simulink model "sim4_5"  (R2022a)
settings: Solver=FixedStepAuto  StartTime=0.0  StopTime=120  FixedStep=0.001  MaxStep=0.002  RelTol=1e-3
libraries: fl_lib x16, nesl_utility x7, dspadpt3 x6, dsparch4 x3
settings Model: Creator=targi  LastModifiedBy=targi

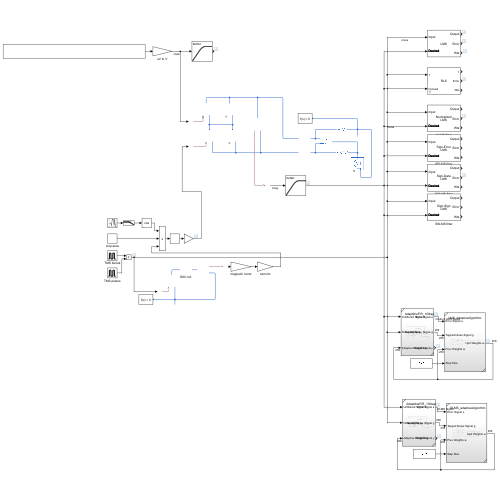
[thumbnail: Simulink's stored preview of the top-level diagram]
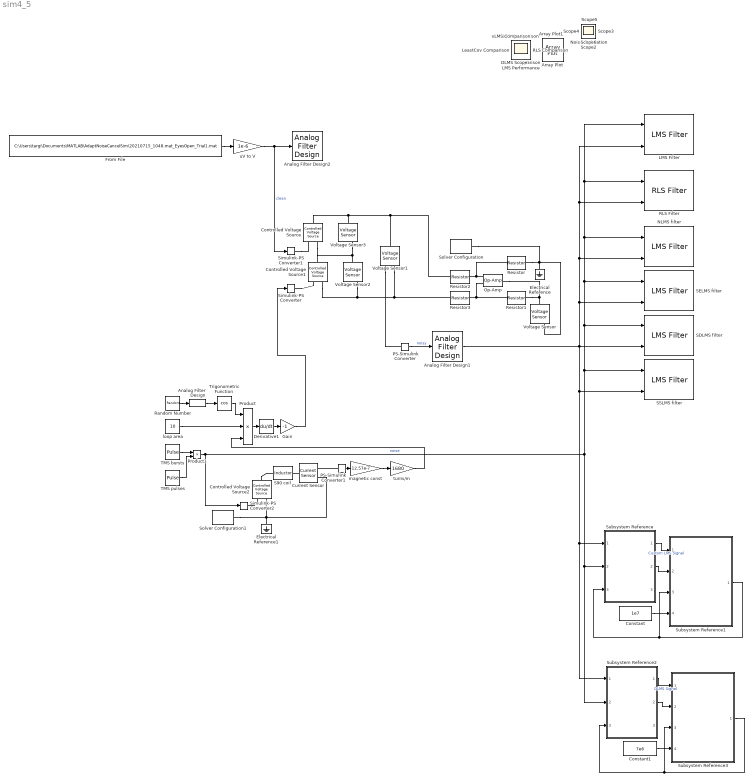
== system sim4_5 ==
  Analog Filter Design : dsparch4/Analog Filter Design  method=Butterworth  filttype=Lowpass  N=8  Wlo=100  Whi=80  Rp=2  Rs=40
  Analog Filter Design1 : dsparch4/Analog Filter Design  method=Butterworth  filttype=Highpass  N=2  Wlo=10  Whi=80  Rp=2  Rs=40
  Analog Filter Design2 : dsparch4/Analog Filter Design  method=Butterworth  filttype=Highpass  N=2  Wlo=10  Whi=80  Rp=2  Rs=40
  Constant : Constant  Value=1e7
  Constant1 : Constant  Value=7e6
  Controlled Voltage Source : fl_lib/Electrical/Electrical Sources/Controlled Voltage Source
      settings: SourceProductBaseCode=PW,SS,VE
  Controlled Voltage Source1 : fl_lib/Electrical/Electrical Sources/Controlled Voltage Source
      settings: SourceProductBaseCode=PW,SS,VE
  Controlled Voltage Source2 : fl_lib/Electrical/Electrical Sources/Controlled Voltage Source
      settings: SourceProductBaseCode=PW,SS,VE
  Current Sensor : fl_lib/Electrical/Electrical Sensors/Current Sensor
      settings: SourceProductBaseCode=PW,SS,VE
  Derivative1 : Derivative
  Electrical Reference : fl_lib/Electrical/Electrical Elements/Electrical Reference
      settings: SourceProductBaseCode=PW,SS,VE
  Electrical Reference1 : fl_lib/Electrical/Electrical Elements/Electrical Reference
      settings: SourceProductBaseCode=PW,SS,VE
  From File : FromFile  FileName=C:\Users\targi\Documents\MATLAB\AdaptNoiseCancelSim\20210715_1048.mat_EyesOpen_Trial1.mat
  Gain : Gain  Gain=-1
  LMS Filter : dspadpt3/LMS Filter  Algo=LMS  L=256  stepflag=Dialog  mu=1e7  leakage=1  ic=0  Adapt=off  resetflag=None  weights=on  addnparflag=off  roundingMode=Floor  overflowMode=off  firstCoeffMode=Binary point scaling  firstCoeffWordLength=16  firstCoeffFracLength=15
      settings: SourceProductBaseCode=DS
  NLMS filter : dspadpt3/LMS Filter  Algo=Normalized LMS  L=256  stepflag=Dialog  mu=1  leakage=1.0  ic=0  Adapt=off  resetflag=None  weights=on  addnparflag=off  roundingMode=Floor  overflowMode=off
      settings: SourceProductBaseCode=DS
  Op-Amp : fl_lib/Electrical/Electrical Elements/Op-Amp  outI_specify=off  outI_priority=None  outI=0 A  outI_nominal_specify=off  outI_nominal_unit=A  outI_nominal_value=1
      settings: SourceProductBaseCode=PW,SS,VE
  PS-Simulink Converter : nesl_utility/PS-Simulink Converter  PhysicalDomain=network_engine_domain  SubClassName=ps_output  LeftPortType=input  RightPortType=output  PseudoPeriodic=off  Frequencies=[]  VectorFormat=inherit  Unit=inherit  AffineConversion=off
      settings: SourceProductBaseCode=SS,PW,VE
  PS-Simulink Converter1 : nesl_utility/PS-Simulink Converter  PhysicalDomain=network_engine_domain  SubClassName=ps_output  LeftPortType=input  RightPortType=output  PseudoPeriodic=off  Frequencies=[]  VectorFormat=inherit  Unit=inherit  AffineConversion=off
      settings: SourceProductBaseCode=SS,PW,VE
  Product : Product  Inputs=3
  Product1 : Product
  RLS Filter : dspadpt3/RLS Filter  L=32  lambdaflag=Dialog  lambda=1  addnparflag=on  ic=0  delta=0.1  Adapt=off  resetflag=None  weights=on
      settings: SourceProductBaseCode=DS
  Random Number : RandomNumber  Variance=.15
  Resistor : fl_lib/Electrical/Electrical Elements/Resistor  R=100 Ohm  i_specify=off  i_priority=None  i=0 A  i_nominal_specify=off  i_nominal_unit=A  i_nominal_value=1  v_specify=off  v_priority=None  v=0 V  v_nominal_specify=off  v_nominal_unit=V  v_nominal_value=1
      settings: SourceProductBaseCode=PW,SS,VE
  Resistor1 : fl_lib/Electrical/Electrical Elements/Resistor  R=100 Ohm  i_specify=off  i_priority=None  i=0 A  i_nominal_specify=off  i_nominal_unit=A  i_nominal_value=1  v_specify=off  v_priority=None  v=0 V  v_nominal_specify=off  v_nominal_unit=V  v_nominal_value=1
      settings: SourceProductBaseCode=PW,SS,VE
  Resistor2 : fl_lib/Electrical/Electrical Elements/Resistor  R=1 Ohm  i_specify=off  i_priority=None  i=0 A  i_nominal_specify=off  i_nominal_unit=A  i_nominal_value=1  v_specify=off  v_priority=None  v=0 V  v_nominal_specify=off  v_nominal_unit=V  v_nominal_value=1
      settings: SourceProductBaseCode=PW,SS,VE
  Resistor3 : fl_lib/Electrical/Electrical Elements/Resistor  R=1 Ohm  i_specify=off  i_priority=None  i=0 A  i_nominal_specify=off  i_nominal_unit=A  i_nominal_value=1  v_specify=off  v_priority=None  v=0 V  v_nominal_specify=off  v_nominal_unit=V  v_nominal_value=1
      settings: SourceProductBaseCode=PW,SS,VE
  S90 coil : fl_lib/Electrical/Electrical Elements/Inductor  l=23.47 uH  r=.01 Ohm  g=1e-9 1/Ohm  i_specify=off  i_priority=None  i=0 A  i_nominal_specify=off  i_nominal_unit=A  i_nominal_value=1  v_specify=off  v_priority=None  v=0 V  v_nominal_specify=off  v_nominal_unit=V  v_nominal_value=1  i_L_specify=off  i_L_priority=High  i_L=0 A  i_L_nominal_specify=off  i_L_nominal_unit=A  i_L_nominal_value=1
      settings: SourceProductBaseCode=PW,SS,VE
  SDLMS filter : dspadpt3/LMS Filter  Algo=Sign-Data LMS  L=256  stepflag=Dialog  mu=1e3  leakage=1.0  ic=0  Adapt=off  resetflag=None  weights=on  addnparflag=off  roundingMode=Floor  overflowMode=off
      settings: SourceProductBaseCode=DS
  SELMS filter : dspadpt3/LMS Filter  Algo=Sign-Error LMS  L=256  stepflag=Dialog  mu=1e4  leakage=1.0  ic=0  Adapt=off  resetflag=None  weights=on  addnparflag=off  roundingMode=Floor  overflowMode=off
      settings: SourceProductBaseCode=DS
  SSLMS filter : dspadpt3/LMS Filter  Algo=Sign-Sign LMS  L=256  stepflag=Dialog  mu=1  leakage=1.0  ic=0  Adapt=off  resetflag=None  weights=on  addnparflag=off  roundingMode=Floor  overflowMode=off
      settings: SourceProductBaseCode=DS
  Simulink-PS Converter : nesl_utility/Simulink-PS Converter  PhysicalDomain=network_engine_domain  SubClassName=ps_input  LeftPortType=input  RightPortType=output  PseudoPeriodic=off  Frequencies=[]  NoiseDistribution=none  NoiseParameters=[]  Unit=1  AffineConversion=off  FilteringAndDerivatives=provide  SimscapeFilterOrder=1  InputFilterTimeConstant=0.001  UdotUserProvided=0
      settings: SourceProductBaseCode=SS,PW,VE
  Simulink-PS Converter1 : nesl_utility/Simulink-PS Converter  PhysicalDomain=network_engine_domain  SubClassName=ps_input  LeftPortType=input  RightPortType=output  PseudoPeriodic=off  Frequencies=[]  NoiseDistribution=none  NoiseParameters=[]  Unit=1  AffineConversion=off  FilteringAndDerivatives=provide  SimscapeFilterOrder=1  InputFilterTimeConstant=0.001  UdotUserProvided=0
      settings: SourceProductBaseCode=SS,PW,VE
  Simulink-PS Converter2 : nesl_utility/Simulink-PS Converter  PhysicalDomain=network_engine_domain  SubClassName=ps_input  LeftPortType=input  RightPortType=output  PseudoPeriodic=off  Frequencies=[]  NoiseDistribution=none  NoiseParameters=[]  Unit=1  AffineConversion=off  FilteringAndDerivatives=provide  SimscapeFilterOrder=1  InputFilterTimeConstant=0.001  UdotUserProvided=0
      settings: SourceProductBaseCode=SS,PW,VE
  Solver Configuration : nesl_utility/Solver Configuration  PhysicalDomain=network_engine_domain  SubClassName=solver  LeftPortType=input  RightPortType=generic  Tones=[]  Harmonics=[]  SimulateNoise=off  Profile=off  UseLocalSampling=off  EnableSwitchedLinearOptims=on  FrequencyDomain=off  UseCCode=off  RelTol=0.001  AbsTol=0.001  MinStep=1e-09  ToWorkspace=off  RevertToSquareIcSolve=off  NumHomotopyIterations=100  PhasorMode=off  PhasorModeNumHarmonics=1  IndexReductionMethod=DerivativeReplacement  DoDC=off  ResidualTolerance=1e-09  UseLocalSolver=off  LocalSolverChoice=NE_BACKWARD_EULER_ADVANCER  LocalSolverSampleTime=0.001  DoFixedCost=off  MaxNonlinIter=3  MaxModeIter=2  ComputeImpulses=off  ImpulseIterations=2  LinearAlgebra=auto  LinearAlgebraNumThread=0  EquationFormulation=NE_TIME_EF  DelaysMemoryBudget=1024  AutomaticFiltering=on  FilteringTimeConstant=0.001  PartitionStorageMethod=AS_NEEDED  PartitionMemoryBudget=1024  PartitionMethod=ROBUST
      settings: SourceProductBaseCode=SS,PW,VE
  Solver Configuration1 : nesl_utility/Solver Configuration  PhysicalDomain=network_engine_domain  SubClassName=solver  LeftPortType=input  RightPortType=generic  Tones=[]  Harmonics=[]  SimulateNoise=off  Profile=off  UseLocalSampling=off  EnableSwitchedLinearOptims=on  FrequencyDomain=off  UseCCode=off  RelTol=0.001  AbsTol=0.001  MinStep=1e-09  ToWorkspace=off  RevertToSquareIcSolve=off  NumHomotopyIterations=100  PhasorMode=off  PhasorModeNumHarmonics=1  IndexReductionMethod=DerivativeReplacement  DoDC=off  ResidualTolerance=1e-09  UseLocalSolver=off  LocalSolverChoice=NE_BACKWARD_EULER_ADVANCER  LocalSolverSampleTime=0.001  DoFixedCost=off  MaxNonlinIter=3  MaxModeIter=2  ComputeImpulses=off  ImpulseIterations=2  LinearAlgebra=auto  LinearAlgebraNumThread=0  EquationFormulation=NE_TIME_EF  DelaysMemoryBudget=1024  AutomaticFiltering=on  FilteringTimeConstant=0.001  PartitionStorageMethod=AS_NEEDED  PartitionMemoryBudget=1024  PartitionMethod=ROBUST
      settings: SourceProductBaseCode=SS,PW,VE
  Subsystem Reference : Subsystem  ReferencedSubsystem=AdaptibleFIR_100taps
  Subsystem Reference1 : Subsystem  ReferencedSubsystem=LMS_adaptiveAlgorithm
  Subsystem Reference2 : Subsystem  ReferencedSubsystem=AdaptibleFIR_100taps
  Subsystem Reference3 : Subsystem  ReferencedSubsystem=DLMS_adaptiveAlgorithm
  TMS bursts : DiscretePulseGenerator  PulseType=Time based  Period=.02  PulseWidth=5
  TMS pulses : DiscretePulseGenerator  PulseType=Time based  Amplitude=1e-4  Period=.2  PulseWidth=29
  Trigonometric Function : Trigonometry  Operator=cos
  Voltage Sensor{,1..3} (4 alike) : fl_lib/Electrical/Electrical Sensors/Voltage Sensor
      settings: SourceProductBaseCode=PW,SS,VE
  loop area : Constant  Value=10
  magnetic const : Gain  Gain=12.57e-7
  turns/m : Gain  Gain=1680
  uV to V : Gain  Gain=1e-6
  Array Plot : ArrayPlot  IOType=viewer  WindowPosition=[698.000000,462.000000,800.000000,500.000000,]  Visible=on  IsFloating=on  ScopeFrameLocation=window  YLimits=[-35.4102,168.2872]  DefaultConfigurationName=dsp.scopes.ArrayPlotBlockSpecification
  Array Plot1 : ArrayPlot  IOType=viewer  WindowPosition=[44.000000,61.000000,800.000000,500.000000,]  Visible=on  IsFloating=on  ScopeFrameLocation=window  YLimits=[-41.2548,164.9494]  DefaultConfigurationName=dsp.scopes.ArrayPlotBlockSpecification
  DLMS Comparison : Scope
  LMS Comparison : Scope
  LMS Performance : Scope
  LeastCov Comparison : Scope
  Noise Estimation : Scope
  RLS Comparison : Scope
  Scope{,1..6} (7 alike) : Scope
  vLMS Comparison : Scope
  wires:
  Product1/1 -> Simulink-PS Converter2/1, RLS Filter/1, LMS Filter/1, NLMS filter/1, SELMS filter/1, SDLMS filter/1, SSLMS filter/1, Subsystem Reference2/2, Subsystem Reference/2  "noise"
  uV to V/1 -> Analog Filter Design2/1, Simulink-PS Converter1/1  "clean"
  PS-Simulink Converter/1 -> Analog Filter Design1/1  "noisy"
  Subsystem Reference/1 -> Subsystem Reference1/1  "Custom LMS Signal"
  Subsystem Reference/2 -> Subsystem Reference1/2
  Subsystem Reference1/1 -> Subsystem Reference1/3, Subsystem Reference/3
  Constant/1 -> Subsystem Reference1/4
  Constant1/1 -> Subsystem Reference3/4
  Subsystem Reference2/2 -> Subsystem Reference3/2
  Subsystem Reference2/1 -> Subsystem Reference3/1  "DLMS Signal"
  Subsystem Reference3/1 -> Subsystem Reference3/3, Subsystem Reference2/3
  loop area/1 -> Product/2
  Trigonometric Function/1 -> Product/1
  Product/1 -> Derivative1/1
  Derivative1/1 -> Gain/1
  Gain/1 -> Simulink-PS Converter/1
  Random Number/1 -> Analog Filter Design/1
  Analog Filter Design/1 -> Trigonometric Function/1
  TMS bursts/1 -> Product1/1
  TMS pulses/1 -> Product1/2
  From File/1 -> uV to V/1
  PS-Simulink Converter1/1 -> magnetic const/1
  magnetic const/1 -> turns/m/1
  turns/m/1 -> Product/3
  Analog Filter Design1/1 -> Subsystem Reference2/1, Subsystem Reference/1, SSLMS filter/2, LMS Filter/2, RLS Filter/2, NLMS filter/2, SELMS filter/2, SDLMS filter/2
  connections:
  Resistor2/RConn1 -- Resistor/LConn1 -- Op-Amp/LConn1
  Resistor1/LConn1 -- Op-Amp/LConn2 -- Resistor3/RConn1
  Op-Amp/RConn1 -- Resistor1/RConn1 -- Voltage Sensor/LConn1
  Resistor/RConn1 -- Solver Configuration/RConn1 -- Electrical Reference/LConn1 -- Voltage Sensor/RConn2
  Resistor2/LConn1 -- Controlled Voltage Source/LConn1 -- Voltage Sensor3/LConn1 -- Voltage Sensor1/LConn1
  Voltage Sensor3/RConn2 -- Controlled Voltage Source/RConn2 -- Controlled Voltage Source1/LConn1 -- Voltage Sensor2/LConn1
  Voltage Sensor1/RConn2 -- Controlled Voltage Source1/RConn2 -- Voltage Sensor2/RConn2 -- Resistor3/LConn1
  Simulink-PS Converter/RConn1 -- Controlled Voltage Source1/RConn1
  Simulink-PS Converter1/RConn1 -- Controlled Voltage Source/RConn1
  Voltage Sensor1/RConn1 -- PS-Simulink Converter/LConn1
  Simulink-PS Converter2/RConn1 -- Controlled Voltage Source2/RConn1
  S90 coil/LConn1 -- Controlled Voltage Source2/LConn1
  S90 coil/RConn1 -- Current Sensor/LConn1
  Current Sensor/RConn2 -- Controlled Voltage Source2/RConn2 -- Electrical Reference1/LConn1 -- Solver Configuration1/RConn1
  PS-Simulink Converter1/LConn1 -- Current Sensor/RConn1
